simulink model "mskTest"  (R2018b)
settings: Solver=VariableStepDiscrete  StartTime=0.0  StopTime=inf  RelTol=1e-3
libraries: commdigbbndcpm2 x2, commrandsrc3 x1, commsink2 x1
settings Model: Creator=Tinchy  LastModifiedBy=Tinchy
settings DataIOCC: LimitDataPoints=on  SaveOutput=off  SaveTime=off
settings OptimizationCC: BooleanDataType=off  DefaultParameterBehavior=Inlined  LocalBlockOutputs=off  LifeSpan=inf
settings DebuggingCC: AlgebraicLoopMsg=error  SingleTaskRateTransMsg=error  AllowSymbolicDim=off  SFUnexpectedBacktrackingDiag=warning  SFNoUnconditionalDefaultTransitionDiag=warning  SFExecutionAtInitializationDiag=none
settings SFSimCC: SimUseLocalCustomCode=off
settings RTWCC: RTWUseLocalCustomCode=off
settings CodeAppCC: StateflowObjectComments=on
settings GRTTargetCC: TargetLangStandard=C89/C90 (ANSI)  GeneratePreprocessorConditionals=Disable all
settings ConfigComp: CovMetricSettings=dw  CovHtmlReporting=on  CovSaveCumulativeToWorkspaceVar=on  CovSaveSingleToWorkspaceVar=on  CovExternalEMLEnable=off  CovSFcnEnable=off

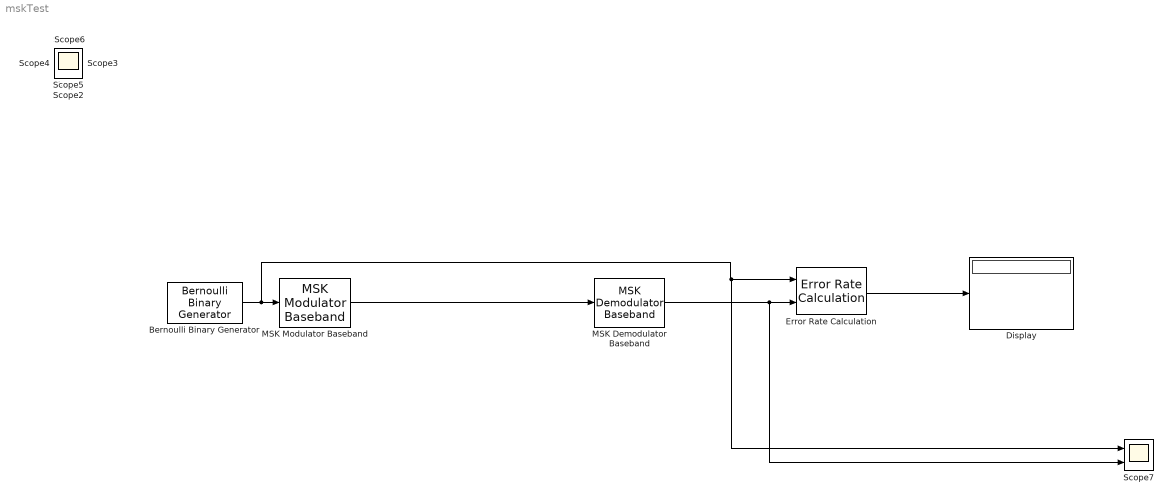
== system mskTest ==
  Bernoulli Binary Generator : commrandsrc3/Bernoulli Binary Generator  ProbabilityOfZero=0.5  SeedSource=Parameter  Seed=124  SampleTime=0.1  SamplesPerFrame=1  OutputDataType=double  SimulateUsing=Interpreted execution
  Display : Display
  Error Rate Calculation : commsink2/Error Rate Calculation  N=0  st_delay=100  cp_mode=Entire frame  subframe=[]  PMode=Port  WsName=ErrorVec  RsMode2=off  stop=off  numErr=100  maxBits=1e6
  MSK Demodulator Baseband : commdigbbndcpm2/MSK Demodulator Baseband  outputType=Bit  phaseOffset=0  samplesPerSymbol=8  RateOptions=Enforce single-rate processing  traceBack=16  outDType=double
      settings: SourceProductName=Communications System Toolbox  SourceProductBaseCode=CM
  MSK Modulator Baseband : commdigbbndcpm2/MSK Modulator Baseband  inputType=Bit  phaseOffset=0  samplesPerSymbol=8  RateOptions=Enforce single-rate processing  outDataType=double
      settings: SourceProductName=Communications System Toolbox  SourceProductBaseCode=CM
  Scope7 : Scope  NumInputPorts=2
  Scope{,1..6} (7 alike) : Scope
  wires:
  Bernoulli Binary Generator/1 -> Scope7/1, Error Rate Calculation/1, MSK Modulator Baseband/1
  MSK Modulator Baseband/1 -> MSK Demodulator Baseband/1
  MSK Demodulator Baseband/1 -> Scope7/2, Error Rate Calculation/2
  Error Rate Calculation/1 -> Display/1
